simulink model "Power_Model"  (R2020a)
settings: Solver=VariableStepAuto  StartTime=0.0  StopTime=10.0  RelTol=1e-3
settings Model: Creator=Ricky  LastModifiedBy=Ricky

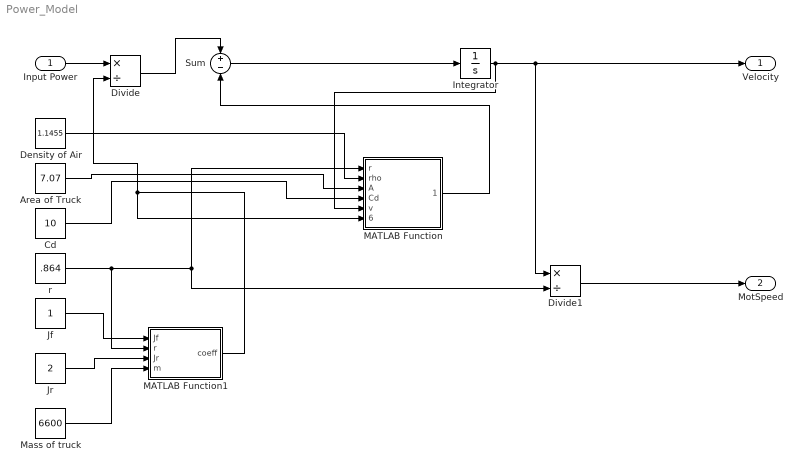
== system Power_Model ==
  Input Power : Inport
  Area of Truck : Constant  Value=7.07
  Cd : Constant  Value=10
  Density of Air : Constant  Value=1.1455
  Divide : Product  Inputs=*/
  Divide1 : Product  Inputs=*/
  Integrator : Integrator
  Jf : Constant
  Jr : Constant  Value=2
  MATLAB Function : MATLAB Function  TreatAsAtomicUnit=on
  MATLAB Function1 : MATLAB Function  TreatAsAtomicUnit=on
  Mass of truck : Constant  Value=6600
  Sum : Sum  Inputs=+-
  r : Constant  Value=.864
  Velocity : Outport
  MotSpeed : Outport  Port=2
  wires:
  Integrator/1 -> MATLAB Function/5(v), Divide1/1, Velocity/1
  Density of Air/1 -> MATLAB Function/2(rho)
  Area of Truck/1 -> MATLAB Function/3(A)
  Cd/1 -> MATLAB Function/4(Cd)
  r/1 -> MATLAB Function1/2(r), MATLAB Function/1(r), Divide1/2
  Mass of truck/1 -> MATLAB Function1/4(m)
  Jr/1 -> MATLAB Function1/3(Jr)
  Jf/1 -> MATLAB Function1/1(Jf)
  MATLAB Function1/1(coeff) -> Divide/2, MATLAB Function/6(inertia_coeff)
  Input Power/1 -> Divide/1
  Divide/1 -> Sum/1
  MATLAB Function/1(Drag_Torque) -> Sum/2
  Sum/1 -> Integrator/1
  Divide1/1 -> MotSpeed/1

== matlab function Power_Model/MATLAB Function1 ==
  data: Jf input; coeff output; r input; Jr input; m input
function coeff= fcn(Jf,r,Jr,m)
out=(Jf/r+Jr+m*r);
coeff=out;

== matlab function Power_Model/MATLAB Function ==
  data: r input; rho input; Drag_Torque output; A input; Cd input; v input; inertia_coeff input
function Drag_Torque = fcn(r,rho,A,Cd,v,inertia_coeff)
coeff=1/2*rho*A*Cd*r/inertia_coeff;
Drag_Torque=coeff*v^2;
